simulink model "simulation"  (R2018b)
settings: Solver=FixedStepDiscrete  StartTime=0.0  StopTime=simtime  FixedStep=stepsize  RelTol=1e-3
undefined symbols (not defined in the file): activate_stop, activate_stop_vmax, ay_stop, Bat_param, deltav_ist, DiscIntNeverNeededParam, EG_wunsch, magnitude, mu_road_LF, mu_road_LR, mu_road_RF, mu_road_RR, par_ASR, par_MDT, par_TIR, par_VEH, select_delta_h, select_M_wheel, stepsize, t, temp_betriebsstrategie, temperature_LTrange, track_left, track_right
libraries: Library_ASK x36, simulink x18, dspstat3 x2, Library_Betriebsstrategie x2, vehicle_model x2, pacejka_trans x1
(part 3 of 6)

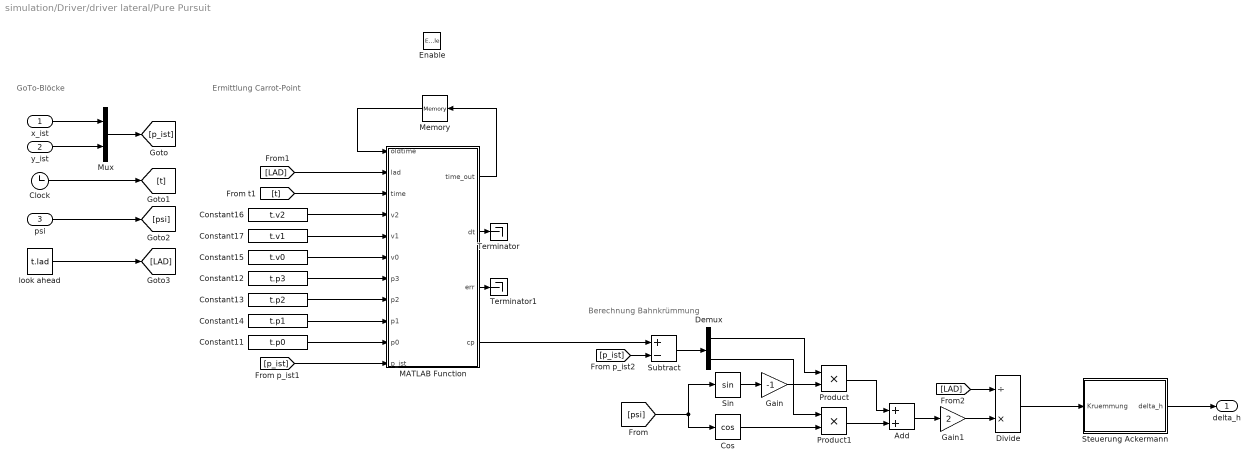
== system simulation/Driver/driver lateral/Pure Pursuit ==
  note: Berechnung Bahnkrümmung
  note: Ermittlung Carrot-Point
  note: GoTo-Blöcke
  x_ist : Inport
  y_ist : Inport  Port=2
  psi : Inport  Port=3
  Enable : EnablePort
  Add : Sum
  Clock : Clock
  Constant11 : Constant  Value=t.p0
  Constant12 : Constant  Value=t.p3
  Constant13 : Constant  Value=t.p2
  Constant14 : Constant  Value=t.p1
  Constant15 : Constant  Value=t.v0
  Constant16 : Constant  Value=t.v2
  Constant17 : Constant  Value=t.v1
  Cos : Trigonometry  Operator=cos
  Demux : Demux  Outputs=2
  Divide : Product  Inputs=/*
  Gain : Gain  Gain=-1
  Gain1 : Gain  Gain=2
  MATLAB Function : MATLAB Function  TreatAsAtomicUnit=on
  Memory : Memory
  Mux : Mux  Inputs=2
  Product : Product
  Product1 : Product
  Sin : Trigonometry
  Steuerung Ackermann : Subsystem
  Subtract : Sum  Inputs=+-
  Terminator : Terminator
  Terminator1 : Terminator
  look ahead : Constant  Value=t.lad
  delta_h : Outport
  wires:
  x_ist/1 -> Mux/1
  y_ist/1 -> Mux/2
  Mux/1 -> [p_ist]
  Clock/1 -> [t]
  psi/1 -> [psi]
  Constant17/1 -> MATLAB Function/5(v1)
  [p_ist] -> MATLAB Function/11(p_ist)
  Memory/1 -> MATLAB Function/1(oldtime)
  Constant16/1 -> MATLAB Function/4(v2)
  Constant15/1 -> MATLAB Function/6(v0)
  Constant14/1 -> MATLAB Function/9(p1)
  [t] -> MATLAB Function/3(time)
  Constant13/1 -> MATLAB Function/8(p2)
  Constant11/1 -> MATLAB Function/10(p0)
  Constant12/1 -> MATLAB Function/7(p3)
  MATLAB Function/1(time_out) -> Memory/1
  [p_ist] -> Subtract/2
  [psi] -> Cos/1, Sin/1
  Subtract/1 -> Demux/1
  MATLAB Function/4(cp) -> Subtract/1
  Cos/1 -> Product1/2
  Sin/1 -> Gain/1
  Demux/1 -> Product/1
  Product/1 -> Add/1
  Product1/1 -> Add/2
  Add/1 -> Gain1/1
  Gain/1 -> Product/2
  Demux/2 -> Product1/1
  Gain1/1 -> Divide/2
  Divide/1 -> Steuerung Ackermann/1(Kruemmung)
  Steuerung Ackermann/1(delta_h) -> delta_h/1
  look ahead/1 -> [LAD]
  [LAD] -> MATLAB Function/2(lad)
  [LAD] -> Divide/1
  MATLAB Function/2(dt) -> Terminator/1
  MATLAB Function/3(err) -> Terminator1/1

== system simulation/Driver/driver lateral/Regler Kreisfahrt ==
  r_ist : Inport
  r_soll : Inport  Port=2
  0 : Constant  Value=0
  Abs : Abs
  Add : Sum  Inputs=+++
  Constant : Constant  Value=par_VEH.l
  Discrete-Time Integrator : DiscreteIntegrator  gainval=1000  SampleTime=-1  ICPrevOutput=DiscIntNeverNeededParam  ICPrevScaledInput=DiscIntNeverNeededParam
  Divide1 : Product  Inputs=*/
  Gain : Gain  Gain=75
  Isteer : Gain  Gain=par_VEH.isteer_skalar
  Logical Operator : Logic  Operator=NOT  Inputs=1  AllPortsSameDT=off  OutDataTypeStr=boolean
  Math Function : Math  Operator=reciprocal  SaturateOnIntegerOverflow=on
  Math Function1 : Math  Operator=reciprocal  SaturateOnIntegerOverflow=on
  Saturation1 : Saturate  UpperLimit=1000  LowerLimit=-1000
  Sum3 : Sum  Inputs=|-+
  Switch1 : Switch  Criteria=u2 > Threshold  Threshold=0.5e-3
  Unit Delay3 : UnitDelay  SampleTime=-1
  not_zero3 : Subsystem
  not_zero4 : Subsystem
  delta_h : Outport
  wires:
  Gain/1 -> Add/2
  Math Function1/1 -> Sum3/2
  not_zero4/1(Out1) -> Math Function1/1
  Unit Delay3/1 -> delta_h/1
  Math Function/1 -> Sum3/1
  Constant/1 -> Divide1/1
  Add/1 -> Unit Delay3/1
  Divide1/1 -> Isteer/1
  Isteer/1 -> Add/3
  r_ist/1 -> not_zero3/1(In1)
  r_soll/1 -> not_zero4/1(In1), Divide1/2
  not_zero3/1(Out1) -> Saturation1/1
  Sum3/1 -> Gain/1, Switch1/3, Abs/1
  Switch1/1 -> Discrete-Time Integrator/1, Logical Operator/1
  0/1 -> Switch1/1
  Discrete-Time Integrator/1 -> Add/1
  Logical Operator/1 -> ?
  Abs/1 -> Switch1/2
  Saturation1/1 -> Math Function/1

== system simulation/Driver/driver lateral/not_zero2 ==
  In1 : Inport
  Constant : Constant  Value=0.0000000000001
  Switch : Switch  Criteria=u2 ~= 0
  Out1 : Outport
  wires:
  In1/1 -> Switch/1, Switch/2
  Constant/1 -> Switch/3
  Switch/1 -> Out1/1

== system simulation/Driver/driver longitudinal/On ==
  Constant : Constant  Value=select_delta_h
  Constant1 : Constant  Value=4
  Relational Operator : RelationalOperator  Operator===  OutDataTypeStr=boolean  RndMeth=Simplest
  On : Outport
  wires:
  Constant/1 -> Relational Operator/1
  Constant1/1 -> Relational Operator/2
  Relational Operator/1 -> On/1

== system simulation/Driver/driver longitudinal/Subsystem ==
  r_stat : Inport
  Add : Sum
  Add1 : Sum
  Bias : Bias  Bias=-2.5/3.6
  Bus Selector : BusSelector  OutputSignals=r_stat_RF,r_stat_LF,r_stat_RR,r_stat_LR
  Constant : Constant  Value=par_MDT.VA.em.nmax
  Constant1 : Constant  Value=60
  Constant10 : Constant  Value=par_MDT.HA.em.nmax
  Constant2 : Constant  Value=par_MDT.VA.trans.i_gears
  Constant3 : Constant  Value=pi
  Constant4 : Constant  Value=2
  Constant6 : Constant  Value=60
  Constant7 : Constant  Value=par_MDT.HA.trans.i_gears
  Constant8 : Constant  Value=pi
  Constant9 : Constant  Value=2
  Divide : Product  Inputs=*//***
  Divide1 : Product  Inputs=**//**
  Gain : Gain  Gain=0.5
  Gain1 : Gain  Gain=0.5
  If : If
  If Action Subsystem : Subsystem  TreatAsAtomicUnit=on
  If Action Subsystem1 : Subsystem  TreatAsAtomicUnit=on
  If Action Subsystem2 : Subsystem  TreatAsAtomicUnit=on
  If Action Subsystem3 : Subsystem  TreatAsAtomicUnit=on
  If1 : If
  Inf : Constant  Value=100000
  Inf1 : Constant  Value=100000
  Merge : Merge
  Merge1 : Merge
  MinMax : MinMax
  Minimum : dspstat3/Minimum  operation=minimum  fcn=Value  indexBase=One  operateOver=Each column  Dimension=1  InputProcessing=Columns as channels (frame based)  reset=None  roiEnable=off  roiType=Rectangles  roiPortion=Entire ROI  roiOutput=Individual statistics for each ROI  roiFlag=off  roundingMode=Floor  overflowMode=off
      settings: SourceProductName=DSP System Toolbox  SourceProductBaseCode=DS
  Minimum1 : dspstat3/Minimum  operation=minimum  fcn=Value  indexBase=One  operateOver=Each column  Dimension=1  InputProcessing=Columns as channels (frame based)  reset=None  roiEnable=off  roiType=Rectangles  roiPortion=Entire ROI  roiOutput=Individual statistics for each ROI  roiFlag=off  roundingMode=Floor  overflowMode=off
      settings: SourceProductName=DSP System Toolbox  SourceProductBaseCode=DS
  Mux : Mux  Inputs=2
  v_max : Outport
  wires:
  Constant2/1 -> Minimum/1
  Minimum/1 -> Divide/2
  Constant1/1 -> Divide/3
  Constant4/1 -> Divide/4
  Constant3/1 -> Divide/5
  Constant7/1 -> Minimum1/1
  Add1/1 -> Gain1/1
  Merge1/1 -> Divide1/2
  Minimum1/1 -> Divide1/3
  Constant6/1 -> Divide1/4
  Constant9/1 -> Divide1/5
  Constant8/1 -> Divide1/6
  r_stat/1 -> Bus Selector/1
  Bus Selector/1 -> Add/1  "<r_stat_RF>"
  Bus Selector/2 -> Add/2  "<r_stat_LF>"
  Bus Selector/3 -> Add1/1  "<r_stat_RR>"
  Bus Selector/4 -> Add1/2  "<r_stat_LR>"
  Gain/1 -> Divide/6
  Add/1 -> Gain/1
  Gain1/1 -> Divide1/1
  Divide/1 -> Mux/1
  Divide1/1 -> Mux/2
  Mux/1 -> MinMax/1
  MinMax/1 -> Bias/1
  Bias/1 -> v_max/1
  Constant/1 -> If Action Subsystem/1(In1), If/1
  If/1 -> If Action Subsystem/Action
  If/2 -> If Action Subsystem1/Action
  Inf/1 -> If Action Subsystem1/1(In1)
  If Action Subsystem/1(Out1) -> Merge/1
  If Action Subsystem1/1(Out1) -> Merge/2
  Merge/1 -> Divide/1
  Inf1/1 -> If Action Subsystem3/1(In1)
  If1/2 -> If Action Subsystem3/Action
  If Action Subsystem3/1(Out1) -> Merge1/2
  Constant10/1 -> If Action Subsystem2/1(In1), If1/1
  If1/1 -> If Action Subsystem2/Action
  If Action Subsystem2/1(Out1) -> Merge1/1

== system simulation/Driver/driver longitudinal/Trajektorienfolge ==
  note: PD-Fehlerregler
  note: Mittlerer Reifenradius
  note: Luftwiderstand
  note: Rollwiderstand
  note: Beschleunigswiderstand
  <a_veh> : Inport
  <p_long> : Inport  Port=2
  v_veh : Inport  Port=3
  r_stat : Inport  Port=4
  Enable : EnablePort
  Add2 : Sum  Inputs=+++
  Add5 : Sum  Inputs=++++
  Bus Selector2 : BusSelector  OutputSignals=r_stat_RF,r_stat_LF,r_stat_RR,r_stat_LR
  Constant1 : Constant  Value=par_VEH.m
  Constant11 : Constant  Value=par_VEH.cx
  Constant12 : Constant  Value=par_VEH.rhoair
  Constant15 : Constant  Value=par_VEH.g
  Constant16 : Constant  Value=par_TIR.QSY1
  Constant2 : Constant  Value=par_VEH.m
  Constant3 : Constant  Value=0.5
  Demux : Demux  Outputs=2
  Gain1 : Gain  Gain=-1
  Gain3 : Gain  Gain=1/4
  Kraft zu Moment : Product
  PID Controller : simulink/Continuous/PID Controller  Controller=PID  Form=Parallel  TimeDomain=Discrete-time  SampleTime=-1  IntegratorMethod=Forward Euler  FilterMethod=Forward Euler  ControllerParametersSource=internal  P=1000  I=0  D=1000  UseFilter=on  N=100  TunerSelectOption=Transfer Function Based (PID Tuner App)  InitialConditionSource=internal  InitialConditionForIntegrator=0  InitialConditionForFilter=0  DifferentiatorICPrevScaledInput=0  ExternalReset=none  TrackingMode=off  Kt=1  LimitOutput=off  UpperSaturationLimit=inf  LowerSaturationLimit=-inf  LinearizeAsGain=on  AntiWindupMode=none  Kb=1  POutMin=[]  POutMax=[]  IOutMin=[]  IOutMax=[]  DOutMin=[]  DOutMax=[]  NOutMin=[]  NOutMax=[]  SumOutMin=[]  SumOutMax=[]  SaturationOutMin=[]  SaturationOutMax=[]  PParamMin=[]  PParamMax=[]  IParamMin=[]  IParamMax=[]  DParamMin=[]  DParamMax=[]  NParamMin=[]  NParamMax=[]  KbParamMin=[]  KbParamMax=[]  KtParamMin=[]  KtParamMax=[]  KbOutMin=[]  KbOutMax=[]  KtOutMin=[]  KtOutMax=[]  IntegratorOutMin=[]  IntegratorOutMax=[]  FilterOutMin=[]  FilterOutMax=[]  SumI1OutMin=[]  SumI1OutMax=[]  SumI2OutMin=[]  SumI2OutMax=[]  SumI3OutMin=[]  SumI3OutMax=[]  SumI4OutMin=[]  SumI4OutMax=[]  SumDOutMin=[]  SumDOutMax=[]  DifferentiatorOutMin=[]  DifferentiatorOutMax=[]  FilterDiffOutCoefMin=[]  FilterDiffOutCoefMax=[]  ReciprocalOutMin=[]  ReciprocalOutMax=[]  SumDenOutMin=[]  SumDenOutMax=[]  SumNumOutMin=[]  SumNumOutMax=[]  DivideOutMin=[]  DivideOutMax=[]  IntegratorContinuousStateAttributes=''  IntegratorStateMustResolveToSignalObject=off  IntegratorRTWStateStorageClass=Auto  FilterContinuousStateAttributes=''  FilterStateMustResolveToSignalObject=off  FilterRTWStateStorageClass=Auto  ParallelPVariant=InternalParameters  IdealPVariant=Disabled  IVariant=InternalParameters  DVariant=InternalParameters  IntegratorVariant=Discrete  SatVariant=Disabled  AWVariant=Passthrough  PCopyVariant=Disabled  TRVariant=Disabled  FdbkBlocksVariant=Forward  IdealPFdbkVariant=Disabled  SatFdbkVariant=Disabled  DerivativeFilterVariant=ForwardEulerFilter  NVariant=InternalParameters  NCopyVariant=Disabled  FilterICVariant=InternalICsFilter  IntegratorICVariant=InternalICs  ExternalResetVariant=Disabled  TRSumVariant=Passthrough  SumFdbkVariant=Disabled  SumVariant=Sum_PID
  Product2 : Product
  Product3 : Product  Inputs=4
  Product6 : Product  Inputs=3
  Scope : Scope
  Sum4 : Sum  Inputs=|++
  Terminator : Terminator
  square : Math  Operator=square  SaturateOnIntegerOverflow=on
  M_Wheel : Outport
  wires:
  Demux/1 -> Product2/2
  Constant1/1 -> Product2/1
  Product2/1 -> Add2/1
  v_veh/1 -> square/1
  square/1 -> Product3/1
  Constant11/1 -> Product3/2
  Constant3/1 -> Product3/4
  Constant12/1 -> Product3/3
  Product3/1 -> Add2/3
  Add2/1 -> Kraft zu Moment/1
  Gain3/1 -> Kraft zu Moment/2
  Product6/1 -> Add2/2
  Constant16/1 -> Product6/2
  Constant15/1 -> Product6/3
  Sum4/1 -> Scope/1, M_Wheel/1
  Kraft zu Moment/1 -> Sum4/1
  <a_veh>/1 -> Demux/1
  Constant2/1 -> Product6/1
  r_stat/1 -> Bus Selector2/1
  Bus Selector2/1 -> Add5/1  "<r_stat_RF>"
  Bus Selector2/3 -> Add5/3  "<r_stat_RR>"
  Bus Selector2/4 -> Add5/4  "<r_stat_LR>"
  Bus Selector2/2 -> Add5/2  "<r_stat_LF>"
  Add5/1 -> Gain3/1
  <p_long>/1 -> Gain1/1
  Demux/2 -> Terminator/1
  PID Controller/1 -> Sum4/2
  Gain1/1 -> PID Controller/1

== system simulation/Vehicle/Antriebsstrang und Radmomentenverteilung/Batterie ==
  P_LE_DC : Inport
  BMS sampletime : Constant  Value=stepsize
  Division : Product  Inputs=/*  SaturateOnIntegerOverflow=on
  Division{1..3,6} (4 alike) : Product  SaturateOnIntegerOverflow=on
  Division4 : Product  Inputs=*/  SaturateOnIntegerOverflow=on
  Division5 : Product  Inputs=/*  SaturateOnIntegerOverflow=on
  Electrical battery cell model : Subsystem
  Initial battery state : UnitDelay  InitialCondition=par_MDT.AUS.batt.Daten_Batteriemodell.x_init  SampleTime=-1
  Initial battery voltage : UnitDelay  InitialCondition=interp1(par_MDT.AUS.batt.Daten_Batteriemodell.BatPara.ECMPara.OCV.ConstantC.SOC,par_MDT.AUS.batt.Daten_Batteriemodell.BatPara.ECMPara.OCV.ConstantC.U_OCV_C25,par_MDT.AUS.batt.Daten_Batteriemodell.x_init(1))  SampleTime=-1
  MATLAB Function2 : MATLAB Function  TreatAsAtomicUnit=on
  MATLAB Function3 : MATLAB Function  TreatAsAtomicUnit=on
  Minus1 : Gain  Gain=-1
  Minus2 : Gain  Gain=-1
  Parallel : Constant  Value=par_MDT.AUS.batt.Cells_parallel
  Product : Product  Inputs=/*
  Serial : Constant  Value=par_MDT.AUS.batt.Cells_serial
  Sum1 : Sum  Inputs=-+
  Zellkapazität : Constant  Value=par_MDT.AUS.batt.Kapazitaet_Zellen
  SOC : Outport
  pv_batt : Outport  Port=2
  C-Rate : Outport  Port=3
  wires:
  Initial battery state/1 -> Electrical battery cell model/1(x_k)
  Electrical battery cell model/2(y) -> Division6/2, Sum1/1, Initial battery voltage/1  "pv_U"
  Electrical battery cell model/1(x_k+1) -> Initial battery state/1
  Division/1 -> MATLAB Function2/1(u)
  Initial battery voltage/1 -> Product/1
  Electrical battery cell model/4(SOC) -> SOC/1  "SOC"
  Division2/1 -> Division/1
  Parallel/1 -> Division2/2
  Serial/1 -> Division6/1, Division1/1, Division2/1
  BMS sampletime/1 -> Electrical battery cell model/3(dt)
  Division4/1 -> C-Rate/1
  Product/1 -> Electrical battery cell model/2(u), Minus2/1
  Zellkapazität/1 -> Division4/2
  Minus1/1 -> Division/2
  Minus2/1 -> Division4/1
  P_LE_DC/1 -> Division5/2, Minus1/1
  Division5/1 -> Division3/2
  Division6/1 -> Division5/1
  Sum1/1 -> Division1/2
  MATLAB Function2/1(y) -> Product/2
  Electrical battery cell model/3(OCV) -> Sum1/2
  Division1/1 -> Division3/1
  Division3/1 -> MATLAB Function3/1(u)
  MATLAB Function3/1(y) -> pv_batt/1

== system simulation/Vehicle/Antriebsstrang und Radmomentenverteilung/Drehzahlrückführung az HA ==
  note: Nur bei AZ und TS wird Block aktiviert
  Aktivator az : Inport
  "i_Gang " : Inport  Port=2
  "Radrehzahlen " : Inport  Port=3
  n_Kupplung_geschlossen_HA : Inport  Port=4
  TS_HA : Inport  Port=5
  Compare To Zero : simulink/Logic and Bit Operations/Compare To Zero  relop=>  OutDataTypeStr=boolean
  Compare To Zero2 : simulink/Logic and Bit Operations/Compare To Zero  relop=>  OutDataTypeStr=boolean
  "Drehzahlrückführung az HA, TS" : Subsystem  AncestorBlock=Library_ASK/Drehzahlrückführung az fuer mmG
      mask Display: set_param(gcb, 'BackgroundColor', '[0.9,0.7,1]');
  "Drehzahlrückführung az HA,OD & eTV " : Subsystem  AncestorBlock=Library_ASK/Drehzahlrückführung az fuer mmG
      mask Display: set_param(gcb, 'BackgroundColor', '[0.9,0.7,1]');
  Logical Operator35 : Logic  AllPortsSameDT=off  OutDataTypeStr=boolean
  Switch : Switch  Criteria=u2 > Threshold
  Verzögerungsglied : Subsystem
  n_motor : Outport
  wires:
  Compare To Zero/1 -> Logical Operator35/2
  Aktivator az/1 -> "Drehzahlrückführung az HA,OD & eTV "/Enable, [az_HA]
  "Radrehzahlen "/1 -> "Drehzahlrückführung az HA,OD & eTV "/1(Raddrehzahlen)
  [TS_HA] -> Switch/2
  "Drehzahlrückführung az HA,OD & eTV "/1(Motordrehzahl) -> Switch/3
  Switch/1 -> n_motor/1
  "Drehzahlrückführung az HA, TS"/1(Motordrehzahl) -> Verzögerungsglied/1(M)
  Verzögerungsglied/1(M_d) -> Switch/1
  [az_HA] -> Compare To Zero2/1
  Compare To Zero2/1 -> Logical Operator35/1
  n_Kupplung_geschlossen_HA/1 -> "Drehzahlrückführung az HA, TS"/2("n_k_geschl ")
  Logical Operator35/1 -> "Drehzahlrückführung az HA, TS"/Enable
  [TS_HA] -> Compare To Zero/1
  "i_Gang "/1 -> "Drehzahlrückführung az HA,OD & eTV "/2(i_Gang), "Drehzahlrückführung az HA, TS"/1(" i_gang ")
  TS_HA/1 -> [TS_HA]

== system simulation/Vehicle/Antriebsstrang und Radmomentenverteilung/Drehzahlrückführung az VA ==
  note: Nur bei AZ und TS wird Block aktiviert
  Aktivator az : Inport
  "i_Gang " : Inport  Port=2
  "Radrehzahlen " : Inport  Port=3
  n_Kupplung_geschlossen_VA : Inport  Port=4
  TS_VA : Inport  Port=5
  Compare To Zero : simulink/Logic and Bit Operations/Compare To Zero  relop=>  OutDataTypeStr=boolean
  Compare To Zero2 : simulink/Logic and Bit Operations/Compare To Zero  relop=>  OutDataTypeStr=boolean
  "Drehzahlrückführung az VA, TS" : Subsystem  AncestorBlock=Library_ASK/Drehzahlrückführung az fuer mmG
      mask Display: set_param(gcb, 'BackgroundColor', '[0.9,0.7,1]');
  "Drehzahlrückführung az VA,OD & eTV " : Subsystem  AncestorBlock=Library_ASK/Drehzahlrückführung az fuer mmG
      mask Display: set_param(gcb, 'BackgroundColor', '[0.9,0.7,1]');
  Logical Operator35 : Logic  AllPortsSameDT=off  OutDataTypeStr=boolean
  Switch : Switch  Criteria=u2 > Threshold
  Verzögerungsglied : Subsystem
  n_motor : Outport
  wires:
  Compare To Zero/1 -> Logical Operator35/2
  Aktivator az/1 -> "Drehzahlrückführung az VA,OD & eTV "/Enable, [az_VA]
  "Radrehzahlen "/1 -> "Drehzahlrückführung az VA,OD & eTV "/1(Raddrehzahlen)
  [TS_VA] -> Switch/2
  "Drehzahlrückführung az VA,OD & eTV "/1(Motordrehzahl) -> Switch/3
  Switch/1 -> n_motor/1
  "Drehzahlrückführung az VA, TS"/1(Motordrehzahl) -> Verzögerungsglied/1(M)
  Verzögerungsglied/1(M_d) -> Switch/1
  [az_VA] -> Compare To Zero2/1
  Compare To Zero2/1 -> Logical Operator35/1
  n_Kupplung_geschlossen_VA/1 -> "Drehzahlrückführung az VA, TS"/2("n_k_geschl ")
  Logical Operator35/1 -> "Drehzahlrückführung az VA, TS"/Enable
  [TS_VA] -> Compare To Zero/1
  "i_Gang "/1 -> "Drehzahlrückführung az VA,OD & eTV "/2(i_Gang), "Drehzahlrückführung az VA, TS"/1(" i_gang ")
  TS_VA/1 -> [TS_VA]

== system simulation/Vehicle/Antriebsstrang und Radmomentenverteilung/PT_HA1 ==
  M : Inport
  IC : InitialCondition  Value=0
  PT1_VA : DiscreteTransferFcn  Numerator=par_VEH.dt.other.PT_Num  Denominator=par_VEH.dt.other.PT_Denom
  Zero-Order Hold : ZeroOrderHold  SampleTime=stepsize
  M_d : Outport
  wires:
  IC/1 -> M_d/1
  PT1_VA/1 -> IC/1
  M/1 -> Zero-Order Hold/1
  Zero-Order Hold/1 -> PT1_VA/1

== system simulation/Vehicle/Antriebsstrang und Radmomentenverteilung/PT_HA2 ==
  M : Inport
  IC : InitialCondition  Value=0
  PT1_VA : DiscreteTransferFcn  Numerator=par_VEH.dt.other.PT_Num  Denominator=par_VEH.dt.other.PT_Denom
  Zero-Order Hold : ZeroOrderHold  SampleTime=stepsize
  M_d : Outport
  wires:
  IC/1 -> M_d/1
  PT1_VA/1 -> IC/1
  M/1 -> Zero-Order Hold/1
  Zero-Order Hold/1 -> PT1_VA/1

== system simulation/Vehicle/Antriebsstrang und Radmomentenverteilung/PT_VA ==
  M : Inport
  IC : InitialCondition  Value=0
  PT1_VA : DiscreteTransferFcn  Numerator=par_VEH.dt.other.PT_Num  Denominator=par_VEH.dt.other.PT_Denom
  Zero-Order Hold : ZeroOrderHold  SampleTime=stepsize
  M_d : Outport
  wires:
  IC/1 -> M_d/1
  PT1_VA/1 -> IC/1
  M/1 -> Zero-Order Hold/1
  Zero-Order Hold/1 -> PT1_VA/1

== system simulation/Vehicle/Antriebsstrang und Radmomentenverteilung/PT_VA1 ==
  M : Inport
  IC : InitialCondition  Value=0
  PT1_VA : DiscreteTransferFcn  Numerator=par_VEH.dt.other.PT_Num  Denominator=par_VEH.dt.other.PT_Denom
  Zero-Order Hold : ZeroOrderHold  SampleTime=stepsize
  M_d : Outport
  wires:
  IC/1 -> M_d/1
  PT1_VA/1 -> IC/1
  M/1 -> Zero-Order Hold/1
  Zero-Order Hold/1 -> PT1_VA/1

== system simulation/Vehicle/Betriebsstrategie/10 Hz Tiefpass ==
  note: https://de.mathworks.com/help/physmod/sps/ref/lowpassfilterdiscreteorcontinuous.html
  In1 : Inport
  Bus Creator : BusCreator  Inputs=4
  Demux : Demux
  Differenzmoment Vorne : Sum  Inputs=+-
  Differenzmoment hinten : Sum  Inputs=+-
  Discrete Filter1 : DiscreteFilter  Numerator=[(stepsize/0.1)]  Denominator=[1 ((stepsize/0.1)-1)]
  Discrete Filter2 : DiscreteFilter  Numerator=[(stepsize/0.1)]  Denominator=[1 ((stepsize/0.1)-1)]
  Gain{,1..3} (4 alike) : Gain  Gain=0.5
  Summenmoment Vorne : Sum
  Summenmoment Vorne1 : Sum
  Summenmoment Vorne2 : Sum  Inputs=+-
  Summenmoment Vorne3 : Sum
  Summenmoment Vorne4 : Sum  Inputs=+-
  Summenmoment hinten : Sum
  Out1 : Outport
  wires:
  Bus Creator/1 -> Out1/1  "M_antr"
  Demux/2 -> Differenzmoment Vorne/2, Summenmoment Vorne/2
  Demux/1 -> Differenzmoment Vorne/1, Summenmoment Vorne/1
  In1/1 -> Demux/1
  Demux/3 -> Summenmoment hinten/1, Differenzmoment hinten/1
  Demux/4 -> Summenmoment hinten/2, Differenzmoment hinten/2
  Differenzmoment hinten/1 -> Discrete Filter2/1
  Summenmoment Vorne/1 -> Gain/1
  Gain/1 -> Summenmoment Vorne2/1, Summenmoment Vorne1/1
  Gain1/1 -> Summenmoment Vorne2/2, Summenmoment Vorne1/2
  Summenmoment Vorne1/1 -> Bus Creator/1
  Summenmoment Vorne2/1 -> Bus Creator/2
  Summenmoment Vorne4/1 -> Bus Creator/4
  Summenmoment Vorne3/1 -> Bus Creator/3
  Gain3/1 -> Summenmoment Vorne3/2, Summenmoment Vorne4/2
  Discrete Filter2/1 -> Gain3/1
  Gain2/1 -> Summenmoment Vorne3/1, Summenmoment Vorne4/1
  Summenmoment hinten/1 -> Gain2/1
  Discrete Filter1/1 -> Gain1/1
  Differenzmoment Vorne/1 -> Discrete Filter1/1

== system simulation/Vehicle/Betriebsstrategie/Momentenverteilung_und_Schaltstrategie1 ==
  M_wheel : Inport
  delta_wheel : Inport  Port=2
  input : Inport  Port=3
  mu_road : Inport  Port=4
  1=Effizienz oder 0=Fahrdynamik : Constant  Value=temp_betriebsstrategie.Betriebsstrategiewahl
  ASR : Subsystem
  Bus Selector3 : BusSelector  OutputSignals=x.vx
  Feedback Controller : Subsystem
  Feedforward Controller : Subsystem
  Gierrate Referenz Berechnung : Subsystem
  Limitierungen gesamt (mit MVS Limits) : Subsystem
  Logical Operator : Logic  Operator=NOT  AllPortsSameDT=off  OutDataTypeStr=boolean
  Memory : Memory
  Momente für die Reibbremse : Subsystem
  Motor Limits : Subsystem
  Radmomentenaufteilung (Effizienz) : Subsystem
  Radmomentenaufteilung (Standardfahrmanöver) : Subsystem
  Reifen Limits : Subsystem
  "Reifenradius " : Subsystem
  Switch : Switch  Criteria=u2 > Threshold
  Switch1 : Switch  Criteria=u2 > Threshold
  adaptive Limiter : Subsystem
  M_antr : Outport
  M_brems : Outport  Port=2
  Schaltstrategie : Outport  Port=3
  wires:
  Bus Selector3/1 -> Momente für die Reibbremse/3(v_x)  "<vx>"
  Momente für die Reibbremse/1(M_brems) -> M_brems/1
  Gierrate Referenz Berechnung/1(Gierrate ref) -> Feedforward Controller/2(Gierrate ref), Feedback Controller/2(Gierrate ref)  "psip_ref"
  input/1 -> Memory/1
  delta_wheel/1 -> Radmomentenaufteilung (Standardfahrmanöver)/5(Delta_wheel), Gierrate Referenz Berechnung/2(delta_wheel)
  Motor Limits/2(M_limit_zentral) -> Limitierungen gesamt (mit MVS Limits)/3(M_limit_zentral)
  Motor Limits/1(M_limit) -> Limitierungen gesamt (mit MVS Limits)/2(M_limit)
  Reifen Limits/1(Fx_limit) -> Limitierungen gesamt (mit MVS Limits)/1(Fx_limit)
  Switch/1 -> Momente für die Reibbremse/1(M_antr), M_antr/1
  Feedback Controller/1(M_z_FB) -> adaptive Limiter/2(M_z_FB)  "M_z_FB"
  Limitierungen gesamt (mit MVS Limits)/1(Fx_limits) -> Radmomentenaufteilung (Effizienz)/1(Fx_limits), ASR/2(Limits_In)
  1=Effizienz oder 0=Fahrdynamik/1 -> Radmomentenaufteilung (Effizienz)/Enable, Logical Operator/1, Switch/2, Switch1/2
  Radmomentenaufteilung (Standardfahrmanöver)/1(M_antr) -> Switch/3
  Logical Operator/1 -> Radmomentenaufteilung (Standardfahrmanöver)/Enable
  Radmomentenaufteilung (Effizienz)/1(M_antr) -> Switch/1
  Radmomentenaufteilung (Standardfahrmanöver)/2(Schaltstrategie_Dyn) -> Switch1/3
  Switch1/1 -> Schaltstrategie/1
  M_wheel/1 -> Radmomentenaufteilung (Effizienz)/3(M_wheel), Momente für die Reibbremse/2(M_wheel), Radmomentenaufteilung (Standardfahrmanöver)/4(M_wheel)
  Radmomentenaufteilung (Effizienz)/2(Schaltstrategie_Eff) -> Switch1/1
  mu_road/1 -> ASR/3(mu_road)
  ASR/1(Limits_Out) -> Radmomentenaufteilung (Standardfahrmanöver)/1(Fx_limits)
  Memory/1 -> Gierrate Referenz Berechnung/1(input), adaptive Limiter/1(Input), Radmomentenaufteilung (Effizienz)/2(Input), Bus Selector3/1, Radmomentenaufteilung (Standardfahrmanöver)/2(Input), ASR/1(Input), "Reifenradius "/1(Input), Feedforward Controller/1(Input), Feedback Controller/1(Input), Reifen Limits/1(Input), Motor Limits/1(Input)
  "Reifenradius "/1(r_stat_avg) -> Limitierungen gesamt (mit MVS Limits)/4("r_stat_avg ")
  adaptive Limiter/1(M_z_desired) -> Radmomentenaufteilung (Standardfahrmanöver)/3(M_z_desired)
  Feedforward Controller/1(M_z_FF) -> adaptive Limiter/3(M_z_FF)

== system simulation/Vehicle/Fahrzeugmodell/Configurable_model ==
  TIR_parameter : Inport
  TIR_scale : Inport  Port=2
  FZG_Parameter : Inport  Port=3
  ENV_v_wind : Inport  Port=4
  ENV_rho_air : Inport  Port=5
  ENV_road_orientation : Inport  Port=6
  ENV_road_mu : Inport  Port=7
  FZG_delta : Inport  Port=8
  M_antr : Inport  Port=9
  M_brems : Inport  Port=10
  reset : Inport  Port=11
  init_pos : Inport  Port=12
  delta_h : Inport  Port=13
  vehicle_model : vehicle_model/vehicle_model  SystemSampleTime=stepsize
  FZG_omega : Outport
  FZG_phi : Outport  Port=2
  FZG_psi : Outport  Port=3
  FZG_theta : Outport  Port=4
  FZG_x : Outport  Port=5
  FZG_y : Outport  Port=6
  FZG_z : Outport  Port=7
  FZG_wheel_Fl : Outport  Port=8
  FZG_wheel_Ml : Outport  Port=9
  FZG_beta : Outport  Port=10
  FZG_wheel_Fs : Outport  Port=11
  FZG_wheel_Ms : Outport  Port=12
  FZG_wheel_Mh : Outport  Port=13
  FZG_rot_0 : Outport  Port=14
  z_wheel : Outport  Port=15
  kappa : Outport  Port=16
  r_dyn : Outport  Port=17
  Fz : Outport  Port=18
  vl : Outport  Port=19
  F0 : Outport  Port=20
  r_stat : Outport  Port=21
  delta_kinematic : Outport  Port=22
  wires:
  TIR_parameter/1 -> vehicle_model/1
  TIR_scale/1 -> vehicle_model/2
  FZG_Parameter/1 -> vehicle_model/3
  ENV_v_wind/1 -> vehicle_model/4
  ENV_rho_air/1 -> vehicle_model/5
  ENV_road_orientation/1 -> vehicle_model/6
  ENV_road_mu/1 -> vehicle_model/7
  FZG_delta/1 -> vehicle_model/8
  M_antr/1 -> vehicle_model/9
  M_brems/1 -> vehicle_model/10
  reset/1 -> vehicle_model/11
  init_pos/1 -> vehicle_model/12
  delta_h/1 -> vehicle_model/13
  vehicle_model/1 -> FZG_omega/1
  vehicle_model/2 -> FZG_phi/1
  vehicle_model/3 -> FZG_psi/1
  vehicle_model/4 -> FZG_theta/1
  vehicle_model/5 -> FZG_x/1
  vehicle_model/6 -> FZG_y/1
  vehicle_model/7 -> FZG_z/1
  vehicle_model/8 -> FZG_wheel_Fl/1
  vehicle_model/9 -> FZG_wheel_Ml/1
  vehicle_model/10 -> FZG_beta/1
  vehicle_model/11 -> FZG_wheel_Fs/1
  vehicle_model/12 -> FZG_wheel_Ms/1
  vehicle_model/13 -> FZG_wheel_Mh/1
  vehicle_model/14 -> FZG_rot_0/1
  vehicle_model/15 -> z_wheel/1
  vehicle_model/16 -> kappa/1
  vehicle_model/17 -> r_dyn/1  "kappa"
  vehicle_model/18 -> Fz/1  "Fz"
  vehicle_model/19 -> vl/1  "vl"
  vehicle_model/20 -> F0/1  "F0"
  vehicle_model/21 -> r_stat/1
  vehicle_model/22 -> delta_kinematic/1

== system simulation/Vehicle/Fahrzeugmodell/IP_implementation ==
  IP_front : Inport
  IP_rear : Inport  Port=2
  TIR_parameter : Inport  Port=3
  Bus Creator1 : BusCreator  Inputs=125
  Bus Creator2 : BusCreator  Inputs=125
  Bus Creator6 : BusCreator  Inputs=2
  Bus Selector1 : BusSelector  OutputSignals=front,rear
  Bus Selector2 : BusSelector  OutputSignals=UNLOADED_RADIUS,FNOMIN,TYRESIDE,VERTICAL_STIFFNESS,BREFF,DREFF,FREFF,FZMIN,FZMAX,CAMMIN,CAMMAX,KPUMIN,KPUMAX,ALPMIN,ALPMAX,LONGVL,VERTICAL_DAMPING,LOADINDEX,PCX1,PDX1,PDX2,PDX3,PEX1,PEX2,PEX3,PEX4,PKX1,PKX2,PKX3,PHX1,PHX2,PVX1,PVX2,RBX1,RBX2,RCX1,REX1,REX2,RHX1,PTX1,PTX2,PTX3,QSX1,QSX2,QSX3,PCY1,PDY1,PDY2,PDY3,PEY1,PEY2,PEY3,PEY4,PKY1,PKY2,PKY3,PHY1,PHY2,PHY3,PVY1,PVY2,PVY3,PVY4,RBY1,RBY2,RBY3,RCY1,REY1,REY2,RHY1,RHY2,RVY1,RVY2,RVY3,RVY4,RVY5,RVY6,PTY1,PTY2,QSY1,QSY2,QSY3,QSY4,QBZ1,QBZ2,QBZ3,QBZ4,QBZ5,QBZ9,QBZ10,QCZ1,QDZ1,QDZ2,QDZ3,QDZ4,QDZ6,QDZ7,QDZ8,QDZ9,QEZ1,QEZ2,QEZ3,QEZ4,QEZ5,QHZ1,QHZ2,QHZ3,QHZ4,SSZ1,SSZ2,SSZ3,SSZ4,QTZ1,MBELT,PIO,PPX1,PPX2,PPX3,PPX4,PPY1,PPY2,PPY3,PPY4,QPZ1
  Bus Selector4 : BusSelector  OutputSignals=UNLOADED_RADIUS,FNOMIN,TYRESIDE,VERTICAL_STIFFNESS,BREFF,DREFF,FREFF,FZMIN,FZMAX,CAMMIN,CAMMAX,KPUMIN,KPUMAX,ALPMIN,ALPMAX,LONGVL,VERTICAL_DAMPING,LOADINDEX,PCX1,PDX1,PDX2,PDX3,PEX1,PEX2,PEX3,PEX4,PKX1,PKX2,PKX3,PHX1,PHX2,PVX1,PVX2,RBX1,RBX2,RCX1,REX1,REX2,RHX1,PTX1,PTX2,PTX3,QSX1,QSX2,QSX3,PCY1,PDY1,PDY2,PDY3,PEY1,PEY2,PEY3,PEY4,PKY1,PKY2,PKY3,PHY1,PHY2,PHY3,PVY1,PVY2,PVY3,PVY4,RBY1,RBY2,RBY3,RCY1,REY1,REY2,RHY1,RHY2,RVY1,RVY2,RVY3,RVY4,RVY5,RVY6,PTY1,PTY2,QSY1,QSY2,QSY3,QSY4,QBZ1,QBZ2,QBZ3,QBZ4,QBZ5,QBZ9,QBZ10,QCZ1,QDZ1,QDZ2,QDZ3,QDZ4,QDZ6,QDZ7,QDZ8,QDZ9,QEZ1,QEZ2,QEZ3,QEZ4,QEZ5,QHZ1,QHZ2,QHZ3,QHZ4,SSZ1,SSZ2,SSZ3,SSZ4,QTZ1,MBELT,PIO,PPX1,PPX2,PPX3,PPX4,PPY1,PPY2,PPY3,PPY4,QPZ1
  TIR_par : Outport
  wires:
  Bus Creator6/1 -> TIR_par/1
  TIR_parameter/1 -> Bus Selector1/1
  Bus Selector1/1 -> Bus Selector2/1  "<front>"
  Bus Selector2/1 -> Bus Creator1/1  "<UNLOADED_RADIUS>"
  Bus Selector2/2 -> Bus Creator1/2  "<FNOMIN>"
  Bus Selector2/3 -> Bus Creator1/3  "<TYRESIDE>"
  Bus Selector2/4 -> Bus Creator1/4  "<VERTICAL_STIFFNESS>"
  Bus Selector2/5 -> Bus Creator1/5  "<BREFF>"
  Bus Selector2/6 -> Bus Creator1/6  "<DREFF>"
  Bus Selector2/7 -> Bus Creator1/7  "<FREFF>"
  Bus Selector2/8 -> Bus Creator1/8  "<FZMIN>"
  Bus Selector2/9 -> Bus Creator1/9  "<FZMAX>"
  Bus Selector2/10 -> Bus Creator1/10  "<CAMMIN>"
  Bus Selector2/11 -> Bus Creator1/11  "<CAMMAX>"
  Bus Selector2/12 -> Bus Creator1/12  "<KPUMIN>"
  Bus Selector2/13 -> Bus Creator1/13  "<KPUMAX>"
  Bus Selector2/14 -> Bus Creator1/14  "<ALPMIN>"
  Bus Selector2/15 -> Bus Creator1/15  "<ALPMAX>"
  Bus Selector2/16 -> Bus Creator1/16  "<LONGVL>"
  Bus Selector2/17 -> Bus Creator1/17  "<VERTICAL_DAMPING>"
  Bus Selector2/18 -> Bus Creator1/18  "<LOADINDEX>"
  Bus Selector2/19 -> Bus Creator1/19  "<PCX1>"
  Bus Selector2/20 -> Bus Creator1/20  "<PDX1>"
  Bus Selector2/21 -> Bus Creator1/21  "<PDX2>"
  Bus Selector2/22 -> Bus Creator1/22  "<PDX3>"
  Bus Selector2/23 -> Bus Creator1/23  "<PEX1>"
  Bus Selector2/24 -> Bus Creator1/24  "<PEX2>"
  Bus Selector2/25 -> Bus Creator1/25  "<PEX3>"
  Bus Selector2/26 -> Bus Creator1/26  "<PEX4>"
  Bus Selector2/27 -> Bus Creator1/27  "<PKX1>"
  Bus Selector2/28 -> Bus Creator1/28  "<PKX2>"
  Bus Selector2/29 -> Bus Creator1/29  "<PKX3>"
  Bus Selector2/30 -> Bus Creator1/30  "<PHX1>"
  Bus Selector2/31 -> Bus Creator1/31  "<PHX2>"
  Bus Selector2/32 -> Bus Creator1/32  "<PVX1>"
  Bus Selector2/33 -> Bus Creator1/33  "<PVX2>"
  Bus Selector2/34 -> Bus Creator1/34  "<RBX1>"
  Bus Selector2/35 -> Bus Creator1/35  "<RBX2>"
  Bus Selector2/36 -> Bus Creator1/36  "<RCX1>"
  Bus Selector2/37 -> Bus Creator1/37  "<REX1>"
  Bus Selector2/38 -> Bus Creator1/38  "<REX2>"
  Bus Selector2/39 -> Bus Creator1/39  "<RHX1>"
  Bus Selector2/40 -> Bus Creator1/40  "<PTX1>"
  Bus Selector2/41 -> Bus Creator1/41  "<PTX2>"
  Bus Selector2/42 -> Bus Creator1/42  "<PTX3>"
  Bus Selector2/43 -> Bus Creator1/43  "<QSX1>"
  Bus Selector2/44 -> Bus Creator1/44  "<QSX2>"
  Bus Selector2/45 -> Bus Creator1/45  "<QSX3>"
  Bus Selector2/46 -> Bus Creator1/46  "<PCY1>"
  Bus Selector2/47 -> Bus Creator1/47  "<PDY1>"
  Bus Selector2/48 -> Bus Creator1/48  "<PDY2>"
  Bus Selector2/49 -> Bus Creator1/49  "<PDY3>"
  Bus Selector2/50 -> Bus Creator1/50  "<PEY1>"
  Bus Selector2/51 -> Bus Creator1/51  "<PEY2>"
  Bus Selector2/52 -> Bus Creator1/52  "<PEY3>"
  Bus Selector2/53 -> Bus Creator1/53  "<PEY4>"
  Bus Selector2/54 -> Bus Creator1/54  "<PKY1>"
  Bus Selector2/55 -> Bus Creator1/55  "<PKY2>"
  Bus Selector2/56 -> Bus Creator1/56  "<PKY3>"
  Bus Selector2/57 -> Bus Creator1/57  "<PHY1>"
  Bus Selector2/58 -> Bus Creator1/58  "<PHY2>"
  Bus Selector2/59 -> Bus Creator1/59  "<PHY3>"
  Bus Selector2/60 -> Bus Creator1/60  "<PVY1>"
  Bus Selector2/61 -> Bus Creator1/61  "<PVY2>"
  Bus Selector2/62 -> Bus Creator1/62  "<PVY3>"
  Bus Selector2/63 -> Bus Creator1/63  "<PVY4>"
  Bus Selector2/64 -> Bus Creator1/64  "<RBY1>"
  Bus Selector2/65 -> Bus Creator1/65  "<RBY2>"
  Bus Selector2/66 -> Bus Creator1/66  "<RBY3>"
  Bus Selector2/67 -> Bus Creator1/67  "<RCY1>"
  Bus Selector2/68 -> Bus Creator1/68  "<REY1>"
  Bus Selector2/69 -> Bus Creator1/69  "<REY2>"
  Bus Selector2/70 -> Bus Creator1/70  "<RHY1>"
  Bus Selector2/71 -> Bus Creator1/71  "<RHY2>"
  Bus Selector2/72 -> Bus Creator1/72  "<RVY1>"
  Bus Selector2/73 -> Bus Creator1/73  "<RVY2>"
  Bus Selector2/74 -> Bus Creator1/74  "<RVY3>"
  Bus Selector2/75 -> Bus Creator1/75  "<RVY4>"
  Bus Selector2/76 -> Bus Creator1/76  "<RVY5>"
  Bus Selector2/77 -> Bus Creator1/77  "<RVY6>"
  Bus Selector2/78 -> Bus Creator1/78  "<PTY1>"
  Bus Selector2/79 -> Bus Creator1/79  "<PTY2>"
  Bus Selector2/80 -> Bus Creator1/80  "<QSY1>"
  Bus Selector2/81 -> Bus Creator1/81  "<QSY2>"
  Bus Selector2/82 -> Bus Creator1/82  "<QSY3>"
  Bus Selector2/83 -> Bus Creator1/83  "<QSY4>"
  Bus Selector2/84 -> Bus Creator1/84  "<QBZ1>"
  Bus Selector2/85 -> Bus Creator1/85  "<QBZ2>"
  Bus Selector2/86 -> Bus Creator1/86  "<QBZ3>"
  Bus Selector2/87 -> Bus Creator1/87  "<QBZ4>"
  Bus Selector2/88 -> Bus Creator1/88  "<QBZ5>"
  Bus Selector2/89 -> Bus Creator1/89  "<QBZ9>"
  Bus Selector2/90 -> Bus Creator1/90  "<QBZ10>"
  Bus Selector2/91 -> Bus Creator1/91  "<QCZ1>"
  Bus Selector2/92 -> Bus Creator1/92  "<QDZ1>"
  Bus Selector2/93 -> Bus Creator1/93  "<QDZ2>"
  Bus Selector2/94 -> Bus Creator1/94  "<QDZ3>"
  Bus Selector2/95 -> Bus Creator1/95  "<QDZ4>"
  Bus Selector2/96 -> Bus Creator1/96  "<QDZ6>"
  Bus Selector2/97 -> Bus Creator1/97  "<QDZ7>"
  Bus Selector2/98 -> Bus Creator1/98  "<QDZ8>"
  Bus Selector2/99 -> Bus Creator1/99  "<QDZ9>"
  Bus Selector2/100 -> Bus Creator1/100  "<QEZ1>"
  Bus Selector2/101 -> Bus Creator1/101  "<QEZ2>"
  Bus Selector2/102 -> Bus Creator1/102  "<QEZ3>"
  Bus Selector2/103 -> Bus Creator1/103  "<QEZ4>"
  Bus Selector2/104 -> Bus Creator1/104  "<QEZ5>"
  Bus Selector2/105 -> Bus Creator1/105  "<QHZ1>"
  Bus Selector2/106 -> Bus Creator1/106  "<QHZ2>"
  Bus Selector2/107 -> Bus Creator1/107  "<QHZ3>"
  Bus Selector2/108 -> Bus Creator1/108  "<QHZ4>"
  Bus Selector2/109 -> Bus Creator1/109  "<SSZ1>"
  Bus Selector2/110 -> Bus Creator1/110  "<SSZ2>"
  Bus Selector2/111 -> Bus Creator1/111  "<SSZ3>"
  Bus Selector2/112 -> Bus Creator1/112  "<SSZ4>"
  Bus Selector2/113 -> Bus Creator1/113  "<QTZ1>"
  Bus Selector2/114 -> Bus Creator1/114  "<MBELT>"
  Bus Selector2/115 -> Bus Creator1/115  "<PIO>"
  Bus Selector2/116 -> Bus Creator1/116  "<PPX1>"
  Bus Selector2/117 -> Bus Creator1/117  "<PPX2>"
  Bus Selector2/118 -> Bus Creator1/118  "<PPX3>"
  Bus Selector2/119 -> Bus Creator1/119  "<PPX4>"
  Bus Selector2/120 -> Bus Creator1/120  "<PPY1>"
  Bus Selector2/121 -> Bus Creator1/121  "<PPY2>"
  Bus Selector2/122 -> Bus Creator1/122  "<PPY3>"
  Bus Selector2/123 -> Bus Creator1/123  "<PPY4>"
  Bus Selector2/124 -> Bus Creator1/124  "<QPZ1>"
  Bus Creator1/1 -> Bus Creator6/1  "front"
  Bus Selector1/2 -> Bus Selector4/1  "<rear>"
  Bus Selector4/1 -> Bus Creator2/1  "<UNLOADED_RADIUS>"
  Bus Selector4/2 -> Bus Creator2/2  "<FNOMIN>"
  Bus Selector4/3 -> Bus Creator2/3  "<TYRESIDE>"
  Bus Selector4/4 -> Bus Creator2/4  "<VERTICAL_STIFFNESS>"
  Bus Selector4/5 -> Bus Creator2/5  "<BREFF>"
  Bus Selector4/6 -> Bus Creator2/6  "<DREFF>"
  Bus Selector4/7 -> Bus Creator2/7  "<FREFF>"
  Bus Selector4/8 -> Bus Creator2/8  "<FZMIN>"
  Bus Selector4/9 -> Bus Creator2/9  "<FZMAX>"
  Bus Selector4/10 -> Bus Creator2/10  "<CAMMIN>"
  Bus Selector4/11 -> Bus Creator2/11  "<CAMMAX>"
  Bus Selector4/12 -> Bus Creator2/12  "<KPUMIN>"
  Bus Selector4/13 -> Bus Creator2/13  "<KPUMAX>"
  Bus Selector4/14 -> Bus Creator2/14  "<ALPMIN>"
  Bus Selector4/15 -> Bus Creator2/15  "<ALPMAX>"
  Bus Selector4/16 -> Bus Creator2/16  "<LONGVL>"
  Bus Selector4/17 -> Bus Creator2/17  "<VERTICAL_DAMPING>"
  Bus Selector4/18 -> Bus Creator2/18  "<LOADINDEX>"
  Bus Selector4/19 -> Bus Creator2/19  "<PCX1>"
  Bus Selector4/20 -> Bus Creator2/20  "<PDX1>"
  Bus Selector4/21 -> Bus Creator2/21  "<PDX2>"
  Bus Selector4/22 -> Bus Creator2/22  "<PDX3>"
  Bus Selector4/23 -> Bus Creator2/23  "<PEX1>"
  Bus Selector4/24 -> Bus Creator2/24  "<PEX2>"
  Bus Selector4/25 -> Bus Creator2/25  "<PEX3>"
  Bus Selector4/26 -> Bus Creator2/26  "<PEX4>"
  Bus Selector4/27 -> Bus Creator2/27  "<PKX1>"
  Bus Selector4/28 -> Bus Creator2/28  "<PKX2>"
  Bus Selector4/29 -> Bus Creator2/29  "<PKX3>"
  Bus Selector4/30 -> Bus Creator2/30  "<PHX1>"
  Bus Selector4/31 -> Bus Creator2/31  "<PHX2>"
  Bus Selector4/32 -> Bus Creator2/32  "<PVX1>"
  Bus Selector4/33 -> Bus Creator2/33  "<PVX2>"
  Bus Selector4/34 -> Bus Creator2/34  "<RBX1>"
  Bus Selector4/35 -> Bus Creator2/35  "<RBX2>"
  Bus Selector4/36 -> Bus Creator2/36  "<RCX1>"
  Bus Selector4/37 -> Bus Creator2/37  "<REX1>"
  Bus Selector4/38 -> Bus Creator2/38  "<REX2>"
  Bus Selector4/39 -> Bus Creator2/39  "<RHX1>"
  Bus Selector4/40 -> Bus Creator2/40  "<PTX1>"
  Bus Selector4/41 -> Bus Creator2/41  "<PTX2>"
  Bus Selector4/42 -> Bus Creator2/42  "<PTX3>"
  Bus Selector4/43 -> Bus Creator2/43  "<QSX1>"
  Bus Selector4/44 -> Bus Creator2/44  "<QSX2>"
  Bus Selector4/45 -> Bus Creator2/45  "<QSX3>"
  Bus Selector4/46 -> Bus Creator2/46  "<PCY1>"
  Bus Selector4/47 -> Bus Creator2/47  "<PDY1>"
  Bus Selector4/48 -> Bus Creator2/48  "<PDY2>"
  Bus Selector4/49 -> Bus Creator2/49  "<PDY3>"
  Bus Selector4/50 -> Bus Creator2/50  "<PEY1>"
  Bus Selector4/51 -> Bus Creator2/51  "<PEY2>"
  Bus Selector4/52 -> Bus Creator2/52  "<PEY3>"
  Bus Selector4/53 -> Bus Creator2/53  "<PEY4>"
  Bus Selector4/54 -> Bus Creator2/54  "<PKY1>"
  Bus Selector4/55 -> Bus Creator2/55  "<PKY2>"
  Bus Selector4/56 -> Bus Creator2/56  "<PKY3>"
  Bus Selector4/57 -> Bus Creator2/57  "<PHY1>"
  Bus Selector4/58 -> Bus Creator2/58  "<PHY2>"
  Bus Selector4/59 -> Bus Creator2/59  "<PHY3>"
  Bus Selector4/60 -> Bus Creator2/60  "<PVY1>"
  Bus Selector4/61 -> Bus Creator2/61  "<PVY2>"
  Bus Selector4/62 -> Bus Creator2/62  "<PVY3>"
  Bus Selector4/63 -> Bus Creator2/63  "<PVY4>"
  Bus Selector4/64 -> Bus Creator2/64  "<RBY1>"
  Bus Selector4/65 -> Bus Creator2/65  "<RBY2>"
  Bus Selector4/66 -> Bus Creator2/66  "<RBY3>"
  Bus Selector4/67 -> Bus Creator2/67  "<RCY1>"
  Bus Selector4/68 -> Bus Creator2/68  "<REY1>"
  Bus Selector4/69 -> Bus Creator2/69  "<REY2>"
  Bus Selector4/70 -> Bus Creator2/70  "<RHY1>"
  Bus Selector4/71 -> Bus Creator2/71  "<RHY2>"
  Bus Selector4/72 -> Bus Creator2/72  "<RVY1>"
  Bus Selector4/73 -> Bus Creator2/73  "<RVY2>"
  Bus Selector4/74 -> Bus Creator2/74  "<RVY3>"
  Bus Selector4/75 -> Bus Creator2/75  "<RVY4>"
  Bus Selector4/76 -> Bus Creator2/76  "<RVY5>"
  Bus Selector4/77 -> Bus Creator2/77  "<RVY6>"
  Bus Selector4/78 -> Bus Creator2/78  "<PTY1>"
  Bus Selector4/79 -> Bus Creator2/79  "<PTY2>"
  Bus Selector4/80 -> Bus Creator2/80  "<QSY1>"
  Bus Selector4/81 -> Bus Creator2/81  "<QSY2>"
  Bus Selector4/82 -> Bus Creator2/82  "<QSY3>"
  Bus Selector4/83 -> Bus Creator2/83  "<QSY4>"
  Bus Selector4/84 -> Bus Creator2/84  "<QBZ1>"
  Bus Selector4/85 -> Bus Creator2/85  "<QBZ2>"
  Bus Selector4/86 -> Bus Creator2/86  "<QBZ3>"
  Bus Selector4/87 -> Bus Creator2/87  "<QBZ4>"
  Bus Selector4/88 -> Bus Creator2/88  "<QBZ5>"
  Bus Selector4/89 -> Bus Creator2/89  "<QBZ9>"
  Bus Selector4/90 -> Bus Creator2/90  "<QBZ10>"
  Bus Selector4/91 -> Bus Creator2/91  "<QCZ1>"
  Bus Selector4/92 -> Bus Creator2/92  "<QDZ1>"
  Bus Selector4/93 -> Bus Creator2/93  "<QDZ2>"
  Bus Selector4/94 -> Bus Creator2/94  "<QDZ3>"
  Bus Selector4/95 -> Bus Creator2/95  "<QDZ4>"
  Bus Selector4/96 -> Bus Creator2/96  "<QDZ6>"
  Bus Selector4/97 -> Bus Creator2/97  "<QDZ7>"
  Bus Selector4/98 -> Bus Creator2/98  "<QDZ8>"
  Bus Selector4/99 -> Bus Creator2/99  "<QDZ9>"
  Bus Selector4/100 -> Bus Creator2/100  "<QEZ1>"
  Bus Selector4/101 -> Bus Creator2/101  "<QEZ2>"
  Bus Selector4/102 -> Bus Creator2/102  "<QEZ3>"
  Bus Selector4/103 -> Bus Creator2/103  "<QEZ4>"
  Bus Selector4/104 -> Bus Creator2/104  "<QEZ5>"
  Bus Selector4/105 -> Bus Creator2/105  "<QHZ1>"
  Bus Selector4/106 -> Bus Creator2/106  "<QHZ2>"
  Bus Selector4/107 -> Bus Creator2/107  "<QHZ3>"
  Bus Selector4/108 -> Bus Creator2/108  "<QHZ4>"
  Bus Selector4/109 -> Bus Creator2/109  "<SSZ1>"
  Bus Selector4/110 -> Bus Creator2/110  "<SSZ2>"
  Bus Selector4/111 -> Bus Creator2/111  "<SSZ3>"
  Bus Selector4/112 -> Bus Creator2/112  "<SSZ4>"
  Bus Selector4/113 -> Bus Creator2/113  "<QTZ1>"
  Bus Selector4/114 -> Bus Creator2/114  "<MBELT>"
  Bus Selector4/115 -> Bus Creator2/115  "<PIO>"
  Bus Selector4/116 -> Bus Creator2/116  "<PPX1>"
  Bus Selector4/117 -> Bus Creator2/117  "<PPX2>"
  Bus Selector4/118 -> Bus Creator2/118  "<PPX3>"
  Bus Selector4/119 -> Bus Creator2/119  "<PPX4>"
  Bus Selector4/120 -> Bus Creator2/120  "<PPY1>"
  Bus Selector4/121 -> Bus Creator2/121  "<PPY2>"
  Bus Selector4/122 -> Bus Creator2/122  "<PPY3>"
  Bus Selector4/123 -> Bus Creator2/123  "<PPY4>"
  Bus Selector4/124 -> Bus Creator2/124  "<QPZ1>"
  Bus Creator2/1 -> Bus Creator6/2  "rear"
  IP_front/1 -> Bus Creator1/125  "IP"
  IP_rear/1 -> Bus Creator2/125  "IP"

== system simulation/Vehicle/Fahrzeugmodell/Lenkübersetzung ==
  note: beim nach rechts Lenken beide
      | Radwinkel negativ
  note: Rechts lenken in Messung/Kennlinien positiv,
      | in Modell umgekehrt
  delta_h : Inport
  Bus Creator : BusCreator  Inputs=4
  Constant : Constant  Value=0
  Constant1 : Constant  Value=0
  Polynomial : Polyval  Coefs=par_VEH.isteer
  Polynomial1 : Polyval  Coefs=par_VEH.isteer
  Unary Minus : UnaryMinus
  Unary Minus1 : UnaryMinus
  delta_wheel : Outport
  wires:
  Bus Creator/1 -> delta_wheel/1
  Constant/1 -> Bus Creator/3  "delta_RR"
  Constant1/1 -> Bus Creator/4  "delta_LR"
  Unary Minus1/1 -> Bus Creator/2  "delta_LF"
  delta_h/1 -> Unary Minus/1, Polynomial/1
  Polynomial/1 -> Bus Creator/1  "delta_RF"
  Unary Minus/1 -> Polynomial1/1
  Polynomial1/1 -> Unary Minus1/1

== system simulation/Driver/driver lateral/Pure Pursuit/Steuerung Ackermann ==
  Kruemmung : Inport
  Constant : Constant  Value=par_VEH.l
  Gain1 : Gain  Gain=0.5
  Isteer : Gain  Gain=15.48
  Product : Product  Inputs=**
  Unit Delay3 : UnitDelay  SampleTime=-1
  delta_h : Outport
  wires:
  Kruemmung/1 -> Product/2
  Unit Delay3/1 -> Gain1/1
  Constant/1 -> Product/1
  Product/1 -> Isteer/1
  Gain1/1 -> delta_h/1
  Isteer/1 -> Unit Delay3/1

== system simulation/Driver/driver lateral/Regler Kreisfahrt/not_zero3 ==
  In1 : Inport
  Constant : Constant  Value=0.0000000000001
  Switch : Switch  Criteria=u2 ~= 0
  Out1 : Outport
  wires:
  In1/1 -> Switch/1, Switch/2
  Constant/1 -> Switch/3
  Switch/1 -> Out1/1

== system simulation/Driver/driver lateral/Regler Kreisfahrt/not_zero4 ==
  In1 : Inport
  Constant : Constant  Value=0.0000000000001
  Switch : Switch  Criteria=u2 ~= 0
  Out1 : Outport
  wires:
  Switch/1 -> Out1/1
  Constant/1 -> Switch/3
  In1/1 -> Switch/2, Switch/1

== system simulation/Driver/driver longitudinal/Subsystem/If Action Subsystem ==
  In1 : Inport
  Action Port : ActionPort  ActionType=then
  Out1 : Outport
  wires:
  In1/1 -> Out1/1

== system simulation/Driver/driver longitudinal/Subsystem/If Action Subsystem1 ==
  In1 : Inport
  Action Port : ActionPort  ActionType=else
  Out1 : Outport
  wires:
  In1/1 -> Out1/1

== system simulation/Driver/driver longitudinal/Subsystem/If Action Subsystem2 ==
  In1 : Inport
  Action Port : ActionPort  ActionType=then
  Out1 : Outport
  wires:
  In1/1 -> Out1/1

== system simulation/Driver/driver longitudinal/Subsystem/If Action Subsystem3 ==
  In1 : Inport
  Action Port : ActionPort  ActionType=else
  Out1 : Outport
  wires:
  In1/1 -> Out1/1

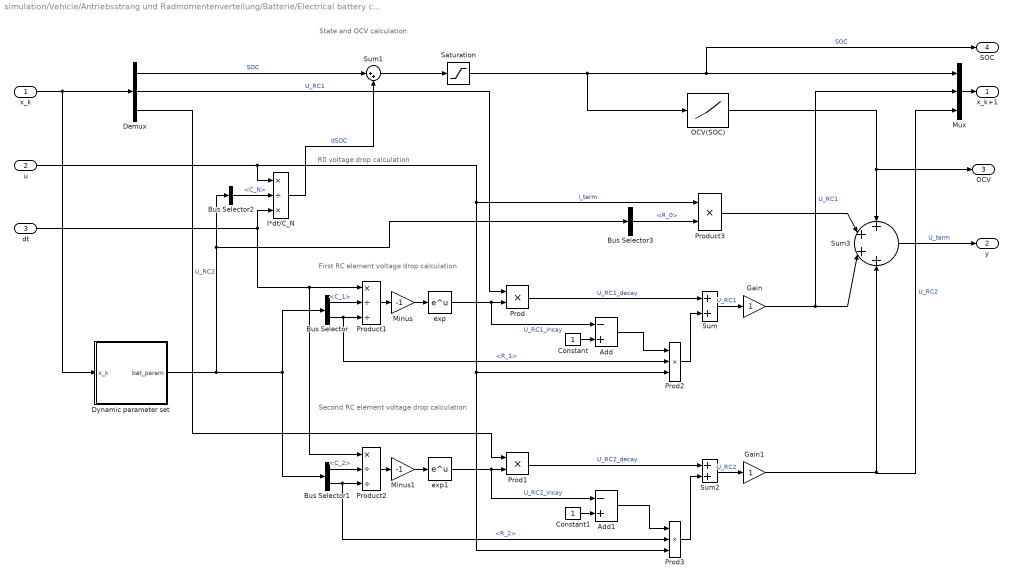
== system simulation/Vehicle/Antriebsstrang und Radmomentenverteilung/Batterie/Electrical battery cell model ==
  note: R0 voltage drop calculation
  note: State and OCV calculation
  note: First RC element voltage drop calculation
  note: Second RC element voltage drop calculation
  x_k : Inport  PortDimensions=[3 1]
  u : Inport  Port=2  PortDimensions=[1 1]
  dt : Inport  Port=3
  Add : Sum  Inputs=-+
  Add1 : Sum  Inputs=-+
  Bus Selector : BusSelector  OutputSignals=C_1,R_1
  Bus Selector1 : BusSelector  OutputSignals=C_2,R_2
  Bus Selector2 : BusSelector  OutputSignals=C_N
  Bus Selector3 : BusSelector  OutputSignals=R_0
  Constant : Constant
  Constant1 : Constant
  Demux : Demux  Outputs=3
  Dynamic parameter set : Subsystem
  Gain : Gain
  Gain1 : Gain
  I*dt/C_N : Product  Inputs=*/*
  Minus : Gain  Gain=-1
  Minus1 : Gain  Gain=-1
  Mux : Mux  Inputs=3
  OCV(SOC) : Lookup_n-D  NumberOfTableDimensions=1  BreakpointsForDimension1=par_MDT.AUS.batt.Daten_Batteriemodell.BatPara.ECMPara.OCV.ConstantC.SOC  Table=par_MDT.AUS.batt.Daten_Batteriemodell.BatPara.ECMPara.OCV.ConstantC.U_OCV_C25  ExtrapMethod=Clip  UseLastTableValue=on  InternalRulePriority=Speed  RndMeth=Simplest  InputSameDT=on
  Prod : Product  Inputs=**
  Prod1 : Product  Inputs=**
  Prod2 : Product  Inputs=***
  Prod3 : Product  Inputs=***
  Product1 : Product  Inputs=*//
  Product2 : Product  Inputs=*//
  Product3 : Product  Inputs=**
  Saturation : Saturate  UpperLimit=1  LowerLimit=0
  Sum : Sum
  Sum1 : Sum  Inputs=|++
  Sum2 : Sum
  Sum3 : Sum  Inputs=++++
  exp : Math  SaturateOnIntegerOverflow=on
  exp1 : Math  SaturateOnIntegerOverflow=on
  x_k+1 : Outport
  y : Outport  Port=2
  OCV : Outport  Port=3
  SOC : Outport  Port=4
  wires:
  Demux/1 -> Sum1/1  "SOC"
  I*dt/C_N/1 -> Sum1/2  "dSOC"
  u/1 -> Prod3/3, Prod2/3, Product3/1, I*dt/C_N/1  "I_term"
  Sum1/1 -> Saturation/1
  Saturation/1 -> Mux/1, SOC/1, OCV(SOC)/1  "SOC"
  Demux/2 -> Prod/1  "U_RC1"
  Dynamic parameter set/1(bat_param) -> Bus Selector/1, Bus Selector1/1, Bus Selector3/1, Bus Selector2/1
  Bus Selector/1 -> Product1/2  "<C_1>"
  Bus Selector/2 -> Prod2/2, Product1/3  "<R_1>"
  Product1/1 -> Minus/1
  Minus/1 -> exp/1
  exp/1 -> Add/1, Prod/2  "U_RC1_incay"
  dt/1 -> I*dt/C_N/3, Product2/1, Product1/1
  Bus Selector1/1 -> Product2/2  "<C_2>"
  Bus Selector1/2 -> Prod3/2, Product2/3  "<R_2>"
  Product2/1 -> Minus1/1
  Minus1/1 -> exp1/1
  exp1/1 -> Add1/1, Prod1/2  "U_RC2_incay"
  Demux/3 -> Prod1/1  "U_RC2"
  Prod1/1 -> Sum2/1  "U_RC2_decay"
  Bus Selector2/1 -> I*dt/C_N/2  "<C_N>"
  Constant/1 -> Add/2
  Constant1/1 -> Add1/2
  Add/1 -> Prod2/1
  Add1/1 -> Prod3/1
  Prod2/1 -> Sum/2
  Prod3/1 -> Sum2/2
  Mux/1 -> x_k+1/1
  Sum/1 -> Gain/1  "U_RC1"
  Sum2/1 -> Gain1/1  "U_RC2"
  Prod/1 -> Sum/1  "U_RC1_decay"
  x_k/1 -> Dynamic parameter set/1(x_k), Demux/1
  Gain/1 -> Mux/2, Sum3/3  "U_RC1"
  Gain1/1 -> Mux/3, Sum3/4  "U_RC2"
  OCV(SOC)/1 -> OCV/1, Sum3/1
  Bus Selector3/1 -> Product3/2  "<R_0>"
  Product3/1 -> Sum3/2
  Sum3/1 -> y/1  "U_term"

== system simulation/Vehicle/Antriebsstrang und Radmomentenverteilung/Drehzahlrückführung az HA/Drehzahlrückführung az HA, TS ==
  note: Das hier ist nur für die az gedacht! Die radnahen kriegen ihre Drehzahlen von den MVS über die from - Blöcke
  " i_gang " : Inport
  "n_k_geschl " : Inport  Port=2
  Enable : EnablePort
  Divide4 : Product  Inputs=**
  Motordrehzahl : Outport
  wires:
  Divide4/1 -> Motordrehzahl/1
  " i_gang "/1 -> Divide4/2
  "n_k_geschl "/1 -> Divide4/1

== system simulation/Vehicle/Antriebsstrang und Radmomentenverteilung/Drehzahlrückführung az HA/Drehzahlrückführung az HA,OD & eTV  ==
  note: Das hier ist nur für die az gedacht! Die radnahen kriegen ihre Drehzahlen von den MVS über die from - Blöcke
  Raddrehzahlen : Inport
  i_Gang : Inport  Port=2
  Enable : EnablePort
  Add11 : Sum
  Demux : Demux  Outputs=2
  Divide4 : Product  Inputs=**
  Gain : Gain  Gain=0.5
  Motordrehzahl : Outport
  wires:
  Demux/1 -> Add11/1
  Raddrehzahlen/1 -> Demux/1
  i_Gang/1 -> Divide4/2
  Add11/1 -> Gain/1
  Demux/2 -> Add11/2
  Divide4/1 -> Motordrehzahl/1
  Gain/1 -> Divide4/1

== system simulation/Vehicle/Antriebsstrang und Radmomentenverteilung/Drehzahlrückführung az HA/Verzögerungsglied ==
  M : Inport
  IC : InitialCondition  Value=0
  PT1_VA : DiscreteTransferFcn  Numerator=par_VEH.dt.other.PT_Num  Denominator=par_VEH.dt.other.PT_Denom
  Zero-Order Hold : ZeroOrderHold  SampleTime=stepsize
  M_d : Outport
  wires:
  IC/1 -> M_d/1
  PT1_VA/1 -> IC/1
  M/1 -> Zero-Order Hold/1
  Zero-Order Hold/1 -> PT1_VA/1

== system simulation/Vehicle/Antriebsstrang und Radmomentenverteilung/Drehzahlrückführung az VA/Drehzahlrückführung az VA, TS ==
  note: Das hier ist nur für die az gedacht! Die radnahen kriegen ihre Drehzahlen von den MVS über die from - Blöcke
  " i_gang " : Inport
  "n_k_geschl " : Inport  Port=2
  Enable : EnablePort
  Divide4 : Product  Inputs=**
  Motordrehzahl : Outport
  wires:
  Divide4/1 -> Motordrehzahl/1
  " i_gang "/1 -> Divide4/2
  "n_k_geschl "/1 -> Divide4/1

== system simulation/Vehicle/Antriebsstrang und Radmomentenverteilung/Drehzahlrückführung az VA/Drehzahlrückführung az VA,OD & eTV  ==
  note: Das hier ist nur für die az gedacht! Die radnahen kriegen ihre Drehzahlen von den MVS über die from - Blöcke
  Raddrehzahlen : Inport
  i_Gang : Inport  Port=2
  Enable : EnablePort
  Add11 : Sum
  Demux : Demux  Outputs=2
  Divide4 : Product  Inputs=**
  Gain : Gain  Gain=0.5
  Motordrehzahl : Outport
  wires:
  Demux/1 -> Add11/1
  Raddrehzahlen/1 -> Demux/1
  i_Gang/1 -> Divide4/2
  Add11/1 -> Gain/1
  Demux/2 -> Add11/2
  Divide4/1 -> Motordrehzahl/1
  Gain/1 -> Divide4/1
